simulink model "modulation_FM"  (R2020a)
settings: Solver=VariableStepAuto  StartTime=0.0  StopTime=1  RelTol=1e-3
settings Model: Creator=kiril_000  LastModifiedBy=kiril_000

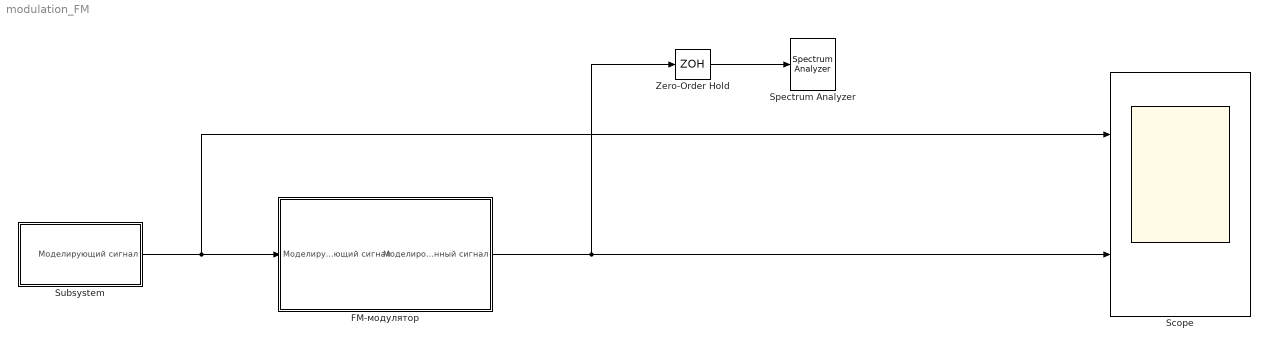
== system modulation_FM ==
  FM-модулятор : Subsystem  mask{m=1000, omega_0=700}
      mask prompts: m "Порядок FM-модуляции"; omega_0 "Частота несущей"
  Scope : Scope  NumInputPorts=2
  Spectrum Analyzer : SpectrumAnalyzer
  Subsystem : Subsystem
  Zero-Order Hold : ZeroOrderHold  SampleTime=1/5000
  wires:
  Subsystem/1(Моделирующий сигнал) -> Scope/1, FM-модулятор/1(Моделирующий сигнал)
  FM-модулятор/1(Моделированный сигнал) -> Scope/2, Zero-Order Hold/1
  Zero-Order Hold/1 -> Spectrum Analyzer/1

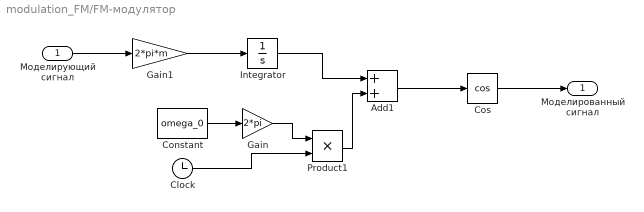
== system modulation_FM/FM-модулятор ==
  Моделирующий сигнал : Inport
  Add1 : Sum
  Clock : Clock
  Constant : Constant  Value=omega_0
  Cos : Trigonometry  Operator=cos
  Gain : Gain  Gain=2*pi
  Gain1 : Gain  Gain=2*pi*m
  Integrator : Integrator
  Product1 : Product
  Моделированный сигнал : Outport
  wires:
  Cos/1 -> Моделированный сигнал/1
  Clock/1 -> Product1/2
  Product1/1 -> Add1/2
  Add1/1 -> Cos/1
  Constant/1 -> Gain/1
  Gain/1 -> Product1/1
  Gain1/1 -> Integrator/1
  Моделирующий сигнал/1 -> Gain1/1
  Integrator/1 -> Add1/1

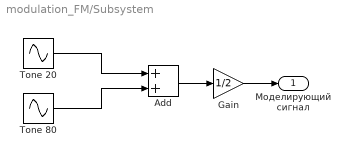
== system modulation_FM/Subsystem ==
  Add : Sum
  Gain : Gain  Gain=1/2
  Tone 20 : Sin  Frequency=2*pi*20  SampleTime=0
  Tone 80 : Sin  Frequency=2*pi*30  SampleTime=0
  Моделирующий сигнал : Outport
  wires:
  Add/1 -> Gain/1
  Tone 80/1 -> Add/2
  Gain/1 -> Моделирующий сигнал/1
  Tone 20/1 -> Add/1
